simulink model "p1_standalone"  (R2014a)
settings: Solver=ode1  SolverMode=SingleTasking  StartTime=0  StopTime=36000  FixedStep=Ts  RelTol=1e-3
PreLoadFcn:
  | InitModel
  | make
InitFcn:
  | InitModel
  | make
values from neighbouring files (symbols this model uses):
  num = num+MTnum(m)    [Build_MtMuMy.m]
  Ts = 0.002    [DSC_Control_Analysis.m]    (also in DSC_Control_Analysis_Exp.m; DSC_Speed_Control_Analysis.m; EC_params_nissan.m; Ext_MPCPara.m = SSD.Ts)
undefined symbols (not defined in the file or in its folder): den, DiscIntNeverNeededParam, gpsins, gr, hal_filter_den, hal_filter_num, Igain_l, Igain_r, Imax_l, Imax_r, Ioff_l, Ioff_r, KB, Kd, KF, Ki, KJ, Kp, param, sglu
libraries: simulink x5, slrtlib x3, xpcdiamondlib x2, UserBlocks x1
(part 1 of 3)
settings Model: SimulationMode=external  ExtModeArmWhenConnect=off  ExtModeAutoUpdateStatusClock=off  Creator=cgadda  LastModifiedBy=cbeal
settings SolverCC: EnableConcurrentExecution=on
settings DataIOCC: LimitDataPoints=off  SignalLogging=off  DSMLogging=off  TimeSaveName=t  OutputSaveName=y  SignalLoggingName=sigsOut
settings OptimizationCC: BooleanDataType=off  InlineParams=on  InlineInvariantSignals=on  ExpressionDepthLimit=2147483647  FoldNonRolledExpr=off  InitFltsAndDblsToZero=on  EfficientFloat2IntCast=on
settings DebuggingCC: SaveWithParameterizedLinksMsg=none  MergeDetectMultiDrivingBlocksExec=error  SolverPrmCheckMsg=none  MultiTaskDSMMsg=warning  MultiTaskCondExecSysMsg=none  StateNameClashWarn=warning
settings HardwareCC: ProdIntDivRoundTo=Zero  ProdEndianess=LittleEndian  ProdHWDeviceType=Generic->32-bit x86 compatible  TargetIntDivRoundTo=Zero  TargetEndianess=LittleEndian  TargetHWDeviceType=32-bit xPC Target (Intel Pentium)
settings RTWCC: SystemTargetFile=slrt.tlc  TemplateMakefile=slrt_default_tmf  Description=Simulink Real-Time  RTWVerbose=off  ProcessScript=slrt_make_rtw_hook  BuildConfiguration=Faster Runs  IncludeERTFirstTime=on  RTWCustomCompilerOptimizations=\Os
settings SimulinkRealTimeCC: GeneratePreprocessorConditionals=Disable all  EnableShiftOperators=on  RL32LogTETModifier=off  RL32LogBufSizeModifier=31000000  xPCRL32EventNumber=100  xPCisDownloadable=off

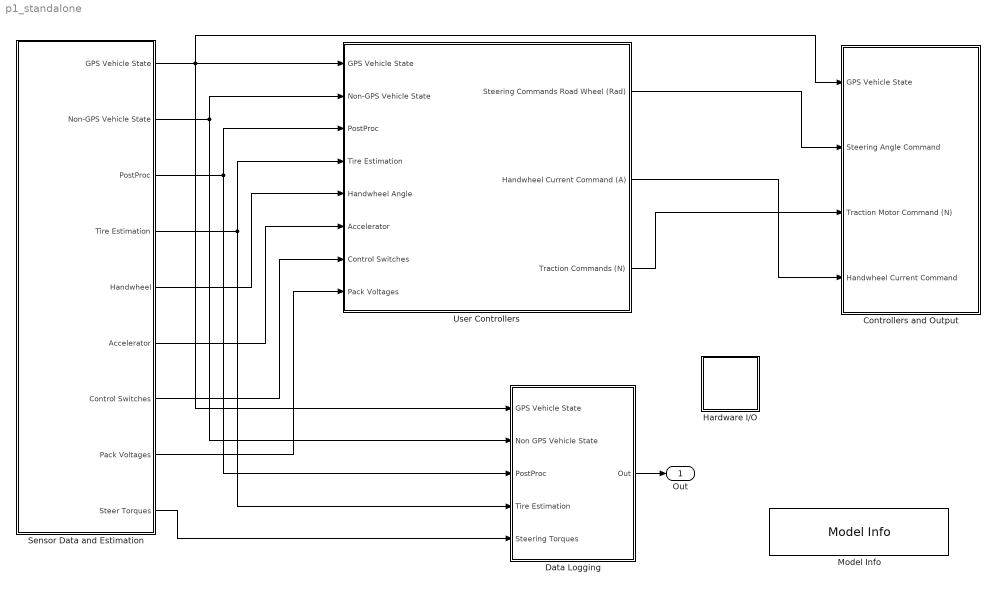
== system p1_standalone ==
  Controllers and Output : Subsystem
  Data Logging : Subsystem
  Hardware I/O : Subsystem  AncestorBlock=HardwareIO/Hardware I//O  mask{OEM4Mode=Velocity (bestvel)}
      mask prompts: OEM4Mode "OEM4 Driver Mode"
      mask init:
      | exist_p1_mdl = sum(strcmp(find_system('p1_standalone', 'searchdepth', 0), 'p1_standalone'));
      | 
      | if (exist_p1_mdl == 1)
      |     set_param('p1_standalone','StopTime','36000');
      |     set_param('p1_standalone','StartTime','0');
      | end
      | 
      | ModeSwitch = [gcs '/Hardware I//O' '/Input' '/OEM4 wgsxyz2enu and status conversion' '/Mode Select'];
      | 
      | if (OEM4Mode == 1)
      |     ModeSelect = 1;
      |     ModeText = 'bestvel';
      |     set_param(ModeSwitch, 'value', '1');
      | elseif (OEM4Mode == 2)
      |     ModeSelect = 0;
      |     ModeText = 'bestxyz';
      |     set_param(ModeSwitch, 'value', '0');
      | end
      mask TypeOptions OEM4Mode: Velocity (bestvel) | Poisition (bestxyz)
      mask Display: disp(['xPC\n' ModeText]);
  Model Info : simulink/Model-Wide Utilities/Model Info  InitialBlockCM=None  BlockCM=None  Frame=off  DisplayStringWithTags=|  HorizontalTextAlignment=Left  LeftAlignmentValue=0.02  SourceBlockDiagram=p1_standalone  TagMaxNumber=20
      | Last saved on: %<LastModificationDate>
      | Save number: %<ModelVersion>
      | Subversion: $Revision: 747 $
  Sensor Data and Estimation : Subsystem
  User Controllers : Subsystem  InitFcn=p1_params SteeringController
  Out : Outport
  wires:
  User Controllers/1(Steering Commands Road Wheel (Rad)) -> Controllers and Output/2(Steering Angle Command)
  Sensor Data and Estimation/1(GPS Vehicle State) -> User Controllers/1(GPS Vehicle State), Controllers and Output/1(GPS Vehicle State), Data Logging/1(GPS Vehicle State)
  Sensor Data and Estimation/2(Non-GPS Vehicle State) -> Data Logging/2(Non GPS Vehicle State), User Controllers/2(Non-GPS Vehicle State)
  Sensor Data and Estimation/3(PostProc) -> User Controllers/3(PostProc), Data Logging/3(PostProc)
  Sensor Data and Estimation/4(Tire Estimation) -> Data Logging/4(Tire Estimation), User Controllers/4(Tire Estimation)
  Data Logging/1(Out) -> Out/1
  User Controllers/3(Traction Commands (N)) -> Controllers and Output/3(Traction Motor Command (N))
  User Controllers/2(Handwheel Current Command (A)) -> Controllers and Output/4(Handwheel Current Command)
  Sensor Data and Estimation/5(Handwheel) -> User Controllers/5(Handwheel Angle)
  Sensor Data and Estimation/6(Accelerator) -> User Controllers/6(Accelerator)
  Sensor Data and Estimation/7(Control Switches) -> User Controllers/7(Control Switches)
  Sensor Data and Estimation/8(Pack Voltages) -> User Controllers/8(Pack Voltages)
  Sensor Data and Estimation/9(Steer Torques) -> Data Logging/5(Steering Torques)

== system p1_standalone/Controllers and Output ==
  GPS Vehicle State : Inport
  Steering Angle Command : Inport  Port=2
  Traction Motor Command (N) : Inport  Port=3
  Handwheel Current Command : Inport  Port=4
  Steering Controller : Subsystem
      mask init:
      | p1_params;
      | SteeringController;
  UI Controller : Subsystem
  tag scope: global_Analog_Meter=global, global_Handwheel_Command=global, global_LED=global, global_Steering_Command=global, global_Traction_Command=global
  wires:
  Steering Angle Command/1 -> Steering Controller/1(Steering Command)
  [global_Handwheel] -> Steering Controller/3(Handwheel Angle)
  [global_Steering] -> Steering Controller/2(Steering Motors)
  [global_Pack_Voltages] -> UI Controller/2(Batteries)
  Steering Controller/1(Current Commands) -> [global_Steering_Command]
  Handwheel Current Command/1 -> [global_Handwheel_Command]
  UI Controller/1(LED) -> [global_LED]
  UI Controller/2(Analog Meter) -> [global_Analog_Meter]
  Traction Motor Command (N)/1 -> [global_Traction_Command]
  GPS Vehicle State/1 -> Steering Controller/4(Vehicle State), UI Controller/1(Vehicle State)
  [global_Cruise_Control] -> UI Controller/3(Switches), Steering Controller/5(switches)

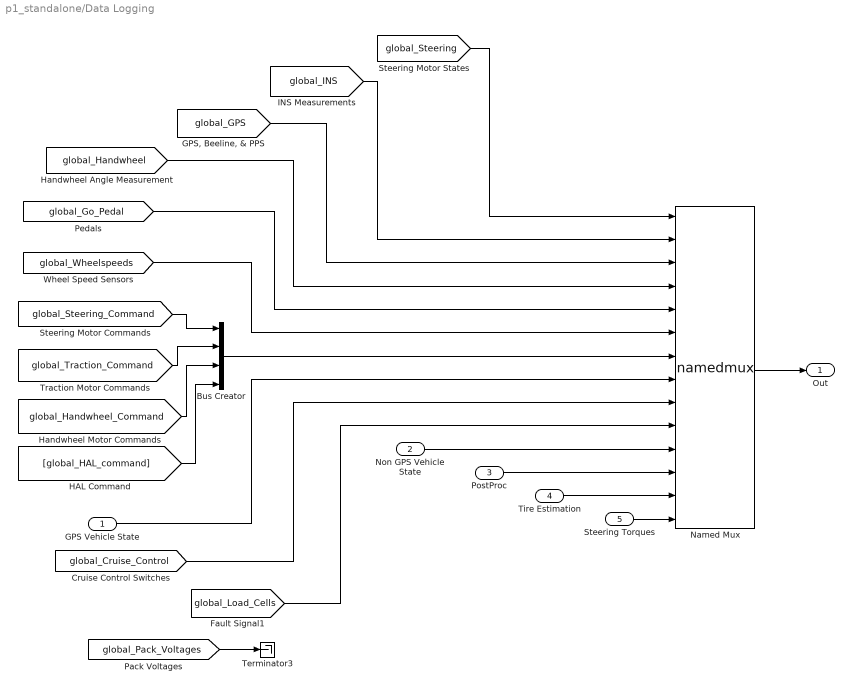
== system p1_standalone/Data Logging ==
  GPS Vehicle State : Inport
  Non GPS Vehicle State : Inport  Port=2
  PostProc : Inport  Port=3
  Tire Estimation : Inport  Port=4
  Steering Torques : Inport  Port=5
  Bus Creator : BusCreator
  Named Mux : S-Function  FunctionName=namedmux  Parameters=inputcount,inputsizes  EnableBusSupport=off  mask{fname=datadesc}
      mask prompts: fname "Data description function name"
      mask help:
      | Combines input signals into a single output vector, according to a structure that provides the names and sizes of each signal.
      |
      | The parameter below should be set to the name of a function which returns a 1xN structure array, where N is the number of input signals.  The structure should contain fields "size" which specifies the width of the input signal, and "name" which specifies its name.
      mask init:
      | desc=eval(fname);
      | %if(class(desc)~='cell')
      | %	error('Incorrect description');
      | %end
      | inputcount=length(desc);
      | if((inputcount<1)|(inputcount>50))
      | 	error('Inappropriate number of inputs.');
      | end
      | 
      | inputsizes=[desc.size];
      | 
      | x=min(inputcount*ones(1,50),1:50);
      mask Display:
      | port_label('input',x(1),desc(x(1)).name);
      | port_label('input',x(2),desc(x(2)).name);
      | port_label('input',x(3),desc(x(3)).name);
      | port_label('input',x(4),desc(x(4)).name);
      | port_label('input',x(5),desc(x(5)).name);
      | port_label('input',x(6),desc(x(6)).name);
      | port_label('input',x(7),desc(x(7)).name);
      | port_label('input',x(8),desc(x(8)).name);
      | port_label('input',x(9),desc(x(9)).name);
      | port_label('input',x(10),desc(x(10)).name);
      | port_label('input',x(11),desc(x(11)).name);
      | port_label('input',x(12),desc(x(12)).name);
      | port_label('input',x(13),desc(x(13)).name);
      | port_label('input',x(14),desc(x(14)).name);
      | port_label('input',x(15),desc(x(15)).name);
      | port_label('input',x(16),desc(x(16)).name);
      | port_label('input',x(17),desc(x(17)).name);
      | port_label('input',x(18),desc(x(18)).name);
      | port_label('input',x(19),desc(x(19)).name);
      | port_label('input',x(20),desc(x(20)).name);
      | port_label('input',x(21),desc(x(21)).name);
      | port_label('input',x(22),desc(x(22)).name);
      | port_label('input',x(23),desc(x(23)).name);
      | port_label('input',x(24),desc(x(24)).name);
      | port_label('input',x(25),desc(x(25)).name);
      | port_label('input',x(26),desc(x(26)).name);
      | port_label('input',x(27),desc(x(27)).name);
      | port_label('input',x(28),desc(x(28)).name);
      | port_label('input',x(29),desc(x(29)).name);
      | port_label('input',x(30),desc(x(30)).name);
  Terminator3 : Terminator
  Out : Outport
  wires:
  GPS Vehicle State/1 -> Named Mux/8
  Named Mux/1 -> Out/1
  [global_Handwheel] -> Named Mux/4
  [global_Steering] -> Named Mux/1
  [global_INS] -> Named Mux/2
  [global_GPS] -> Named Mux/3
  [global_Wheelspeeds] -> Named Mux/6
  [global_Cruise_Control] -> Named Mux/9
  [global_Pack_Voltages] -> Terminator3/1
  [global_Traction_Command] -> Bus Creator/2
  [global_Handwheel_Command] -> Bus Creator/3
  Bus Creator/1 -> Named Mux/7
  [global_Load_Cells] -> Named Mux/10
  [global_Steering_Command] -> Bus Creator/1
  [global_Go_Pedal] -> Named Mux/5
  Non GPS Vehicle State/1 -> Named Mux/11
  PostProc/1 -> Named Mux/12
  Tire Estimation/1 -> Named Mux/13
  Steering Torques/1 -> Named Mux/14
  [global_HAL_command] -> Bus Creator/4

== system p1_standalone/Hardware I//O ==
  Ground : Ground
  Ground1 : Ground
  Input : Subsystem
  Output : Subsystem
  tag scope: global_Cruise_Control=global, global_GPS=global, global_Go_Pedal=global, global_Handwheel=global, global_INS=global, global_Load_Cells=global, global_Pack_Voltages=global, global_Prerecorded_Steering_Command=global, global_Simulation=global, global_Steering=global, global_Wheelspeeds=global
  wires:
  Ground1/1 -> [global_Simulation]
  Ground/1 -> [global_Prerecorded_Steering_Command]
  Input/7(Cruise Control) -> [global_Cruise_Control]
  Input/6(Wheel Speed Sensors) -> [global_Wheelspeeds]
  Input/5(Beeline & GPS) -> [global_GPS]
  Input/4(Go Pedal) -> [global_Go_Pedal]
  Input/3(INS) -> [global_INS]
  Input/2(Steering Motors) -> [global_Steering]
  Input/1(Handwheel) -> [global_Handwheel]
  [global_LED] -> Output/5(Status LED Value)
  [global_Handwheel_Command] -> Output/2(Force Feedback Motor Command)
  [global_Steering_Command] -> Output/1(Steering Motor Commands)
  [global_Analog_Meter] -> Output/4(Analog Meter Command)
  [global_Traction_Command] -> Output/3(Traction Motor Commands (N))
  Input/8(Load Cells) -> [global_Load_Cells]
  Input/9(Pack Voltages) -> [global_Pack_Voltages]

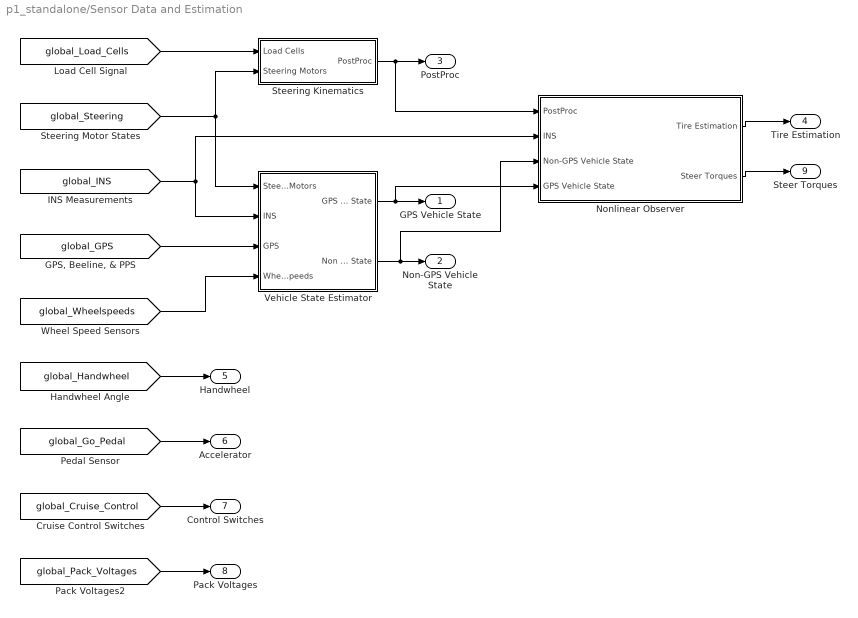
== system p1_standalone/Sensor Data and Estimation ==
  Nonlinear Observer : Subsystem
      mask init:
      | p1_params
      | nissan_steer_lookup_data
      | If_alpha_params
      | [filterb,filtera]=butter(5,0.02);
      | 
      | % dryasphalt = 1;
      | % gravel = 2;
      | % 
      | % AtShoreline = [gcs '/Nonlinear Observer' '/Enable Shoreline Gravel'];
      | % 
      | % % default is dryasphalt
      | % set_param(AtShoreline, 'value', '0');
      | % 
      | % % if gravel selected, make constant AtShoreline = 1
      | % if (roadsurface == gravel)
      | %     set_param(AtShoreline, 'value', '1');
      | % end
      | %
  Steering Kinematics : Subsystem
      mask init:
      | p1_params
      | nissan_steer_lookup_data
  Vehicle State Estimator : Subsystem
      mask init:
      | p1_params;
      | InitVehicleEstimator;
  GPS Vehicle State : Outport
  Non-GPS Vehicle State : Outport  Port=2
  PostProc : Outport  Port=3
  Tire Estimation : Outport  Port=4
  Handwheel : Outport  Port=5
  Accelerator : Outport  Port=6
  Control Switches : Outport  Port=7
  Pack Voltages : Outport  Port=8
  Steer Torques : Outport  Port=9
  wires:
  Vehicle State Estimator/1(GPS Vehicle State) -> GPS Vehicle State/1, Nonlinear Observer/4(GPS Vehicle State)
  Vehicle State Estimator/2(Non GPS Vehicle State) -> Non-GPS Vehicle State/1, Nonlinear Observer/3(Non-GPS Vehicle State)
  Steering Kinematics/1(PostProc) -> PostProc/1, Nonlinear Observer/1(PostProc)
  Nonlinear Observer/1(Tire Estimation) -> Tire Estimation/1
  [global_GPS] -> Vehicle State Estimator/3(GPS)
  [global_INS] -> Vehicle State Estimator/2(INS), Nonlinear Observer/2(INS)
  [global_Steering] -> Steering Kinematics/2(Steering Motors), Vehicle State Estimator/1(Steering Motors)
  [global_Load_Cells] -> Steering Kinematics/1(Load Cells)
  [global_Wheelspeeds] -> Vehicle State Estimator/4(Wheel Speeds)
  [global_Handwheel] -> Handwheel/1
  [global_Go_Pedal] -> Accelerator/1
  [global_Cruise_Control] -> Control Switches/1
  [global_Pack_Voltages] -> Pack Voltages/1
  Nonlinear Observer/2(Steer Torques) -> Steer Torques/1

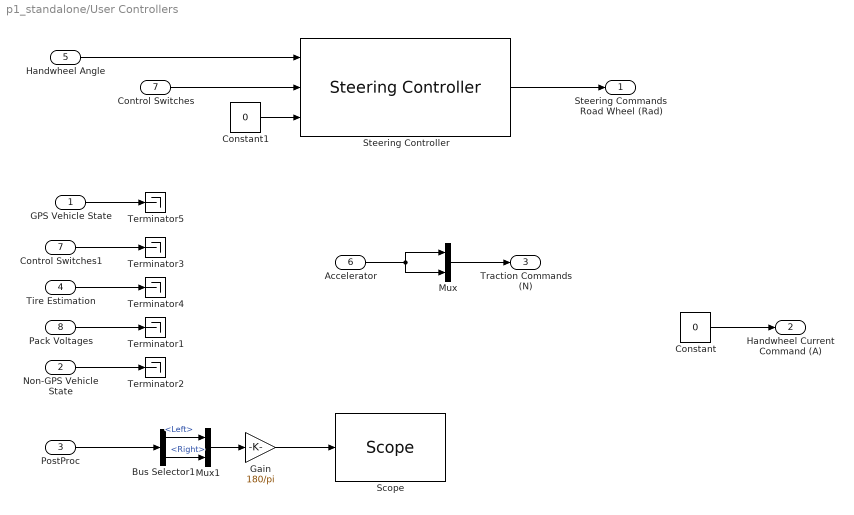
== system p1_standalone/User Controllers ==
  GPS Vehicle State : Inport
  Non-GPS Vehicle State : Inport  Port=2
  PostProc : Inport  Port=3
  Tire Estimation : Inport  Port=4
  Handwheel Angle : Inport  Port=5
  Accelerator : Inport  Port=6
  Control Switches : Inport  Port=7
  Pack Voltages : Inport  Port=8
  Bus Selector1 : BusSelector  OutputSignals=Steer Angles.Left,Steer Angles.Right
  Constant : Constant  Value=0
  Constant1 : Constant  Value=0
  Control Switches1 : InportShadow  Port=7
  Gain : Gain  Gain=180/pi
  Mux : Mux  Inputs=2
  Mux1 : Mux  Inputs=2
  "Scope " : slrtlib/Displays and Logging/Scope   scopeno=2  scopetype=Target  autostart=on  viewmode=Numerical  formatstr='%15.6f'  grid=on  ylimits=[0,0]  nosamples=250  noprepostsamples=0  interleave=1  triggermode=FreeRun  triggersignal=1  trigsignalfromport=off  triggerlevel=0.0  triggerslope=Either  triggerscope=1  triggersample=0  filename=data.dat  mode=Lazy  writesize=512  autorestart=off  dynamicfilemode=off  maxwritefilesize=512*1024^2
  Steering Controller : UserBlocks/Steering Controller  SystemSampleTime=-1
  Terminator{1..5} (5 alike) : Terminator
  Steering Commands Road Wheel (Rad) : Outport
  Handwheel Current Command (A) : Outport  Port=2
  Traction Commands (N) : Outport  Port=3
  wires:
  Non-GPS Vehicle State/1 -> Terminator2/1
  Pack Voltages/1 -> Terminator1/1
  Constant/1 -> Handwheel Current Command (A)/1
  PostProc/1 -> Bus Selector1/1
  Control Switches/1 -> Steering Controller/2
  Handwheel Angle/1 -> Steering Controller/1
  Constant1/1 -> Steering Controller/3
  Mux/1 -> Traction Commands (N)/1
  Accelerator/1 -> Mux/2, Mux/1
  Bus Selector1/1 -> Mux1/1  "<Left>"
  Bus Selector1/2 -> Mux1/2  "<Right>"
  Mux1/1 -> Gain/1
  Steering Controller/1 -> Steering Commands Road Wheel (Rad)/1
  Gain/1 -> "Scope "/1
  Tire Estimation/1 -> Terminator4/1
  Control Switches1/1 -> Terminator3/1
  GPS Vehicle State/1 -> Terminator5/1

== system p1_standalone/Controllers and Output/Steering Controller ==
  Steering Command : Inport
  Steering Motors : Inport  Port=2
  Handwheel Angle : Inport  Port=3
  Vehicle State : Inport  Port=4
  switches : Inport  Port=5
  Bus Selector1 : BusSelector  OutputSignals=Primary
  Bus Selector2 : BusSelector  OutputSignals=Angles
  Bus Selector3 : BusSelector  OutputSignals=Vx
  Bus Selector4 : BusSelector  OutputSignals=Auto-Steer Switch
  Constant : Constant  Value=0
  Demux : Demux  Outputs=2
  Demux1 : Demux  Outputs=2
  LF steering controller : Subsystem
  Mux : Mux  Inputs=2
  Product : Product  SaturateOnIntegerOverflow=on  OutDataTypeStr=Inherit: Same as first input
  RF steering controller : Subsystem
  "Scope " : slrtlib/Displays and Logging/Scope   scopeno=3  scopetype=Target  autostart=on  viewmode=Numerical  formatstr='%15.6f'  grid=on  ylimits=[0,0]  nosamples=250  noprepostsamples=0  interleave=1  triggermode=FreeRun  triggersignal=1  trigsignalfromport=off  triggerlevel=0.0  triggerslope=Either  triggerscope=1  triggersample=0  filename=data.dat  mode=Lazy  writesize=512  autorestart=off  dynamicfilemode=off  maxwritefilesize=512*1024^2
  Steering Geometry & Gearbox Correction : Subsystem
      mask init:
      | p1_params
      | nissan_steer_lookup_data
  standby : Subsystem
  Current Commands : Outport
  wires:
  Vehicle State/1 -> Bus Selector3/1
  Demux1/2 -> RF steering controller/2(actual angle)
  Demux1/1 -> LF steering controller/2(actual angle)
  Demux/1 -> LF steering controller/1(command angle)
  Demux/2 -> RF steering controller/1(command angle)
  RF steering controller/1(current command) -> Mux/2  "Right Current Command"
  Mux/1 -> Product/1
  Steering Motors/1 -> Bus Selector2/1
  Bus Selector2/1 -> Demux1/1  "<Angles>"
  Steering Geometry & Gearbox Correction/1(Shaft Angles) -> Demux/1
  standby/1(Enable) -> Product/2
  Product/1 -> Current Commands/1, "Scope "/1
  Bus Selector3/1 -> standby/2(Speed)  "<Vx>"
  Constant/1 -> RF steering controller/3(aligning moment), LF steering controller/3(aligning moment)
  Steering Command/1 -> Steering Geometry & Gearbox Correction/1(Steer Angles)
  Handwheel Angle/1 -> Bus Selector1/1
  Bus Selector1/1 -> standby/1(Handwheel Angle)  "<Primary>"
  switches/1 -> Bus Selector4/1
  Bus Selector4/1 -> standby/3(autoSteerSwitch)  "<Auto-Steer Switch>"
  LF steering controller/1(current command) -> Mux/1  "Left Current Command"

== system p1_standalone/Controllers and Output/UI Controller ==
  Vehicle State : Inport
  Batteries : Inport  Port=2
  Switches : Inport  Port=3
  Heartbeat Signal : DiscretePulseGenerator  PulseType=Time based  Period=.5  PulseWidth=50
  Speedometer : Subsystem  mask{fsv=25, units=m/s}
      mask prompts: fsv "Full-scale value"
      mask init:
      | unitLabels={'m/s','MPH','KPH'};
      | unitValues={1,2.23693629,3.6};
      | 
      | label=unitLabels{units};
      | scaleFactor=unitValues{units}/fsv;
      mask TypeOptions units: m/s | MPH | KPH
      mask Display: disp(sprintf('%d %s',fsv,label));
  Terminator : Terminator
  Terminator1 : Terminator
  LED : Outport
  Analog Meter : Outport  Port=2
  wires:
  Heartbeat Signal/1 -> LED/1
  Batteries/1 -> Terminator/1
  Vehicle State/1 -> Speedometer/1(Vehicle State)
  Speedometer/1(Meter) -> Analog Meter/1
  Switches/1 -> Terminator1/1

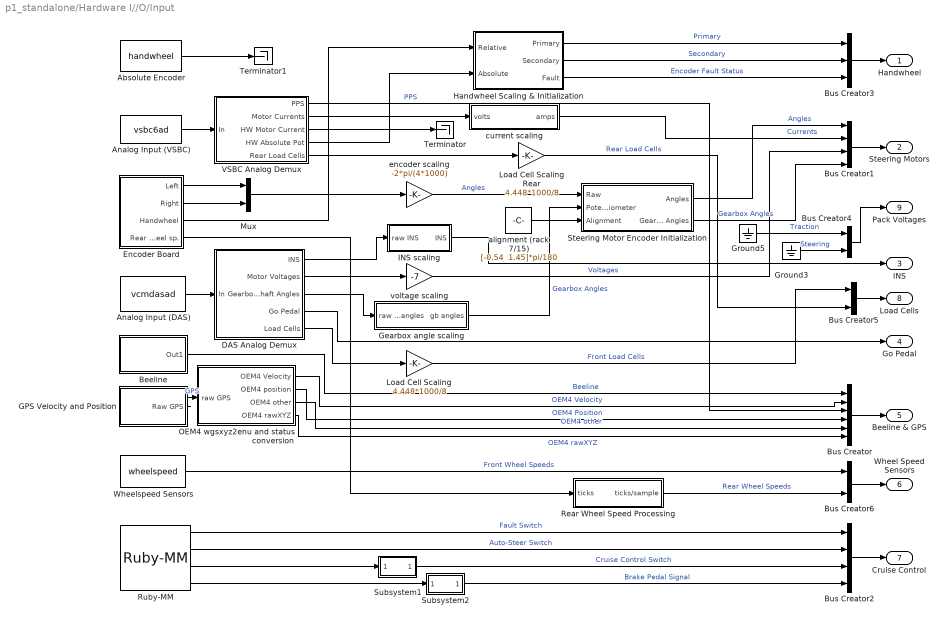
== system p1_standalone/Hardware I//O/Input ==
  Absolute Encoder : S-Function  FunctionName=handwheel  Parameters=Ts  EnableBusSupport=off
  Analog Input (DAS) : S-Function  FunctionName=vcmdasad  Parameters=numChannels, inputVec, sampleTime  EnableBusSupport=off  mask{numChannels=16, inputVec=[4 4 4 4 4 4 4 4 4 4 4 4 4 4 4 4], sampleTime=Ts}
      mask prompts: sampleTime "sample_time"
  Analog Input (VSBC) : S-Function  FunctionName=vsbc6ad  Parameters=numChannels,inpRange,sampTime  EnableBusSupport=off  mask{numChannels=8, inpRange=[4 4 1 4 4 3 3 2], sampTime=Ts}
      mask prompts: numChannels "Number of Channels"; inpRange "Analog Input Range (1: +5; 2: +10; 3: +-5; 4: +-10)"; sampTime "Sampling Time"
  Beeline : Subsystem
      mask Display: disp('beeline');
  Bus Creator : BusCreator  Inputs=6
  Bus Creator1 : BusCreator
  Bus Creator2 : BusCreator
  Bus Creator3 : BusCreator  Inputs=3
  Bus Creator4 : BusCreator  Inputs=2
  Bus Creator5 : BusCreator  Inputs=2
  Bus Creator6 : BusCreator  Inputs=2
  DAS Analog Demux : Subsystem
  Encoder Board : Subsystem
  GPS Velocity and Position : Subsystem
      mask Display: disp('OEM4');
  Gearbox angle scaling : Subsystem
  Ground3 : Ground
  Ground5 : Ground
  Handwheel Scaling & Initialization : Subsystem
  INS scaling : Subsystem
  Load Cell Scaling : Gain  Gain=4.448*1000/8  SaturateOnIntegerOverflow=on  OutDataTypeStr=Inherit: Same as input  ParamDataTypeStr=Inherit: Same as input
  Load Cell Scaling Rear : Gain  Gain=4.448*1000/8  SaturateOnIntegerOverflow=on  OutDataTypeStr=Inherit: Same as input  ParamDataTypeStr=Inherit: Same as input
  Mux : Mux  Inputs=2
  OEM4 wgsxyz2enu and status conversion : Subsystem  AncestorBlock=IOlib/Hardware I//O/Input/INS scaling
  Rear Wheel Speed Processing : Subsystem
  Ruby-MM : xpcdiamondlib/Digital Input/Ruby-MM   channel=[5 6 7 8]  port=A  chip=1  sampletime=Ts  baseaddress=0x300
  Steering Motor Encoder Initialization : Subsystem
      mask init:
      | p1_params
  Subsystem1 : Subsystem
      mask Display: disp('!');
  Subsystem2 : Subsystem
      mask Display: disp('!');
  Terminator : Terminator
  Terminator1 : Terminator
  VSBC Analog Demux : Subsystem
  Wheelspeed Sensors : S-Function  FunctionName=wheelspeed  Parameters=Ts  EnableBusSupport=off
  alignment (rack 7/15) : Constant  Value="[-0.54  1.45]*pi/180"
  current scaling : Subsystem
  encoder scaling : Gain  Gain=-2*pi/(4*1000)  SaturateOnIntegerOverflow=on  OutDataTypeStr=Inherit: Same as input  ParamDataTypeStr=Inherit: Same as input
  voltage scaling : Gain  Gain=-7  SaturateOnIntegerOverflow=on  OutDataTypeStr=Inherit: Same as input  ParamDataTypeStr=Inherit: Same as input
  Handwheel : Outport
  Steering Motors : Outport  Port=2
  INS : Outport  Port=3
  Go Pedal : Outport  Port=4
  Beeline & GPS : Outport  Port=5
  Wheel Speed Sensors : Outport  Port=6
  Cruise Control : Outport  Port=7
  Load Cells : Outport  Port=8
  Pack Voltages : Outport  Port=9
  wires:
  VSBC Analog Demux/4(HW Absolute Pot) -> Handwheel Scaling & Initialization/2(Absolute)
  Handwheel Scaling & Initialization/1(Primary) -> Bus Creator3/1  "Primary"
  OEM4 wgsxyz2enu and status conversion/3(OEM4 other) -> Bus Creator/5  "OEM4 other"
  OEM4 wgsxyz2enu and status conversion/2(OEM4 position) -> Bus Creator/4  "OEM4 Position"
  GPS Velocity and Position/1(Raw GPS) -> OEM4 wgsxyz2enu and status conversion/1(raw GPS)  "GPS"
  OEM4 wgsxyz2enu and status conversion/1(OEM4 Velocity) -> Bus Creator/2  "OEM4 Velocity"
  Ground5/1 -> Bus Creator4/1  "Traction"
  Ruby-MM/1 -> Bus Creator2/1  "Fault Switch"
  Ruby-MM/2 -> Bus Creator2/2  "Auto-Steer Switch"
  Ruby-MM/4 -> Subsystem2/1(In1)
  Ruby-MM/3 -> Subsystem1/1(In1)
  Steering Motor Encoder Initialization/2(Gearbox Angles) -> Bus Creator1/4  "Gearbox Angles"
  alignment (rack 7/15)/1 -> Steering Motor Encoder Initialization/3(Alignment)
  Steering Motor Encoder Initialization/1(Angles) -> Bus Creator1/1  "Angles"
  Handwheel Scaling & Initialization/3(Fault) -> Bus Creator3/3  "Encoder Fault Status"
  encoder scaling/1 -> Steering Motor Encoder Initialization/1(Raw)  "Angles"
  Subsystem2/1(Out1) -> Bus Creator2/4  "Brake Pedal Signal"
  Subsystem1/1(Out1) -> Bus Creator2/3  "Cruise Control Switch"
  Gearbox angle scaling/1(gb angles) -> Steering Motor Encoder Initialization/2(Potentiometer)  "Gearbox Angles"
  DAS Analog Demux/3(Gearbox Shaft Angles) -> Gearbox angle scaling/1(raw gb angles)
  Analog Input (DAS)/1 -> DAS Analog Demux/1(In)
  DAS Analog Demux/1(INS) -> INS scaling/1(raw INS)
  INS scaling/1(INS) -> INS/1
  current scaling/1(amps) -> Bus Creator1/2  "Currents"
  VSBC Analog Demux/2(Motor Currents) -> current scaling/1(volts)
  Bus Creator1/1 -> Steering Motors/1
  Bus Creator/1 -> Beeline & GPS/1
  Beeline/1(Out1) -> Bus Creator/1  "Beeline"
  VSBC Analog Demux/1(PPS) -> Bus Creator/3  "PPS"
  Analog Input (VSBC)/1 -> VSBC Analog Demux/1(In)
  Encoder Board/1(Left) -> Mux/1
  Encoder Board/2(Right) -> Mux/2
  Mux/1 -> encoder scaling/1
  voltage scaling/1 -> Bus Creator1/3  "Voltages"
  DAS Analog Demux/2(Motor Voltages) -> voltage scaling/1
  Bus Creator2/1 -> Cruise Control/1
  DAS Analog Demux/4(Go Pedal) -> Go Pedal/1
  Bus Creator3/1 -> Handwheel/1
  Handwheel Scaling & Initialization/2(Secondary) -> Bus Creator3/2  "Secondary"
  DAS Analog Demux/5(Load Cells) -> Load Cell Scaling/1
  Bus Creator4/1 -> Pack Voltages/1
  Ground3/1 -> Bus Creator4/2  "Steering"
  Encoder Board/3(Handwheel) -> Handwheel Scaling & Initialization/1(Relative)
  VSBC Analog Demux/3(HW Motor Current) -> Terminator/1
  Absolute Encoder/1 -> Terminator1/1
  Load Cell Scaling/1 -> Bus Creator5/1  "Front Load Cells"
  VSBC Analog Demux/5(Rear Load Cells) -> Load Cell Scaling Rear/1
  Load Cell Scaling Rear/1 -> Bus Creator5/2  "Rear Load Cells"
  Bus Creator5/1 -> Load Cells/1
  Wheelspeed Sensors/1 -> Bus Creator6/1  "Front Wheel Speeds"
  Rear Wheel Speed Processing/1(ticks/sample) -> Bus Creator6/2  "Rear Wheel Speeds"
  Encoder Board/4(Rear wheel sp.) -> Rear Wheel Speed Processing/1(ticks)
  Bus Creator6/1 -> Wheel Speed Sensors/1
  OEM4 wgsxyz2enu and status conversion/4(OEM4 rawXYZ) -> Bus Creator/6  "OEM4 rawXYZ"

== system p1_standalone/Hardware I//O/Output ==
  Steering Motor Commands : Inport
  Force Feedback Motor Command : Inport  Port=2
  Traction Motor Commands (N) : Inport  Port=3
  Analog Meter Command : Inport  Port=4
  Status LED Value : Inport  Port=5
  1.0 = full scale : Gain  Gain=9.7  SaturateOnIntegerOverflow=on  OutDataTypeStr=Inherit: Same as input  ParamDataTypeStr=Inherit: Same as input
  ConvertForce2Volt : Subsystem  TreatAsAtomicUnit=on
  Demux : Demux  Outputs=2
  Demux1 : Demux  Outputs=2
  Ground2 : Ground
  "Ruby-MM " : xpcdiamondlib/D//A/Ruby-MM   channel=[1 2 3 4 5 6 7]  range0=+-10  range1=+-10  reset=[1 1 1 1 1 1 1]  initValue=[0 0 0 0 0 0 0]  st=Ts  baseaddress=0x300
  Status LED : S-Function  FunctionName=vsbc8led  EnableBusSupport=off
  amps to volts : Gain  Gain=1/3.96  SaturateOnIntegerOverflow=on  OutDataTypeStr=Inherit: Same as input  ParamDataTypeStr=Inherit: Same as input
  raw signal : Gain  Gain=2  SaturateOnIntegerOverflow=on  OutDataTypeStr=Inherit: Same as input  ParamDataTypeStr=Inherit: Same as input
  saturation : Saturate  UpperLimit=11  LowerLimit=0
  saturation 2 : Saturate  UpperLimit=6  LowerLimit=0  OutDataTypeStr=Inherit: Inherit via back propagation
  saturation1 : Saturate  UpperLimit=2  LowerLimit=-2
  voltage gain : Gain  Gain=7.57/30  SaturateOnIntegerOverflow=on  OutDataTypeStr=Inherit: Same as input  ParamDataTypeStr=Inherit: Same as input
  wires:
  saturation1/1 -> amps to volts/1
  Analog Meter Command/1 -> 1.0 = full scale/1
  Traction Motor Commands (N)/1 -> ConvertForce2Volt/1(ForceDesired)
  Demux1/1 -> "Ruby-MM "/5
  Status LED Value/1 -> Status LED/1
  Demux/1 -> "Ruby-MM "/1
  Demux/2 -> "Ruby-MM "/2
  Ground2/1 -> "Ruby-MM "/4
  1.0 = full scale/1 -> saturation/1
  voltage gain/1 -> Demux/1
  Steering Motor Commands/1 -> voltage gain/1
  Demux1/2 -> "Ruby-MM "/6
  saturation/1 -> "Ruby-MM "/7
  saturation 2/1 -> Demux1/1
  raw signal/1 -> saturation 2/1
  Force Feedback Motor Command/1 -> saturation1/1
  amps to volts/1 -> "Ruby-MM "/3
  ConvertForce2Volt/1(VoltDesired) -> raw signal/1

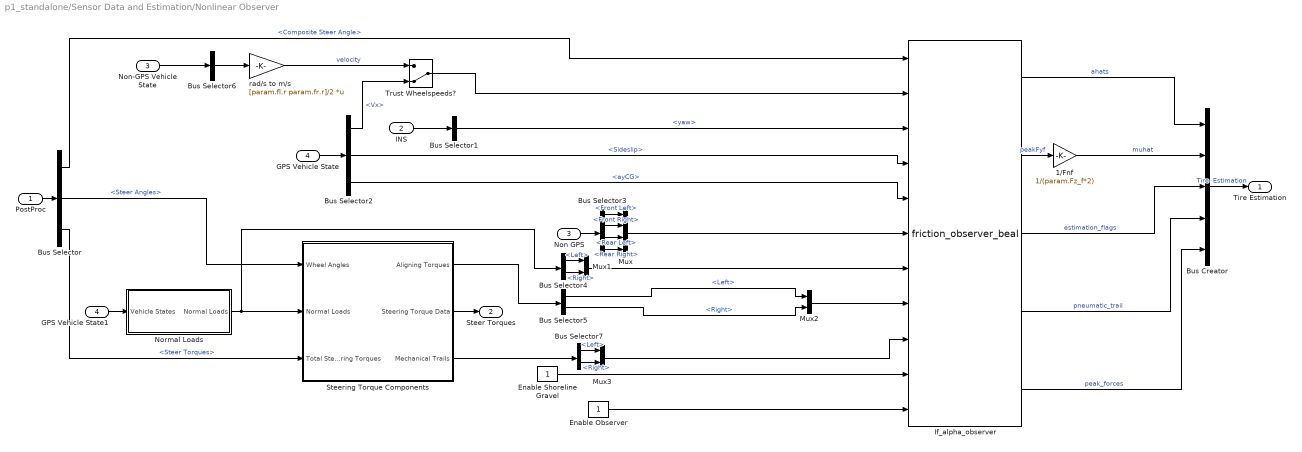
== system p1_standalone/Sensor Data and Estimation/Nonlinear Observer ==
  PostProc : Inport
  INS : Inport  Port=2
  Non-GPS Vehicle State : Inport  Port=3
  GPS Vehicle State : Inport  Port=4
  1/Fnf : Gain  Gain=1/(param.Fz_f*2)
  Bus Creator : BusCreator  Inputs=5
  Bus Selector : BusSelector  OutputSignals=Composite Steer Angle,Steer Angles,Steer Torques
  Bus Selector1 : BusSelector  OutputSignals=yaw
  Bus Selector2 : BusSelector  OutputSignals=Vx,Sideslip,ayCG
  Bus Selector3 : BusSelector  OutputSignals=Wheel Speeds.Front Left,Wheel Speeds.Front Right,Wheel Speeds.Rear Left,Wheel Speeds.Rear Right
  Bus Selector4 : BusSelector  OutputSignals=Left,Right
  Bus Selector5 : BusSelector  OutputSignals=Left,Right
  Bus Selector6 : BusSelector  OutputSignals=Wheel Speeds.Front Left,Wheel Speeds.Front Right  OutputAsBus=on
  Bus Selector7 : BusSelector  OutputSignals=Left,Right
  Enable Observer : Constant
  Enable Shoreline Gravel : Constant
  GPS Vehicle State1 : InportShadow  Port=4
  If_alpha_observer : S-Function  FunctionName=friction_observer_beal  Parameters=Ts, param.a, param.b, param.m, param.Iz, Ifalphaparam.tp0L, Ifalphaparam.tp0R, Ifalphaparam.Caf, Ifalphaparam.Car, Ifalphaparam.Caf_shoreline_sf, Ifalphaparam.Car_shoreline_sf, Ifalphaparam.alphafoffset, Ifalphaparam.alpharoffset, Ifalphaparam.mu_peak_nom, Ifalphaparam.Kaf0, Ifalphaparam.Kaf_sf_Shoreline, Ifalphaparam.Kaf_sf_asphalt, Ifalphaparam.Vfloor, Ifalphaparam.ayfloor, Ifalphaparam.alpha_thres, Ifalphaparam.afhatceil, Ifalphaparam.kappaceil  EnableBusSupport=off
  Mux : Mux
  Mux1 : Mux  Inputs=2
  Mux2 : Mux  Inputs=2
  Mux3 : Mux  Inputs=2
  Non GPS : InportShadow  Port=3
  Normal Loads : Subsystem
      mask init:
      | p1_params
      | nissan_steer_lookup_data
  Steering Torque Components : Subsystem
      mask init:
      | p1_params;
      | nissan_steer_lookup_data;
      | SteeringController;
  Trust Wheelspeeds? : ManualSwitch  CurrentSetting=0
  rad/s to m/s : Gain  Gain=[param.fl.r param.fr.r]/2  Multiplication=Matrix(K*u)
  Tire Estimation : Outport
  Steer Torques : Outport  Port=2
  wires:
  PostProc/1 -> Bus Selector/1
  Bus Creator/1 -> Tire Estimation/1  "Tire  Estimation"
  INS/1 -> Bus Selector1/1
  Non-GPS Vehicle State/1 -> Bus Selector6/1
  rad/s to m/s/1 -> Trust Wheelspeeds?/1  "velocity"
  Bus Selector/1 -> If_alpha_observer/1  "<Composite Steer Angle>"
  Bus Selector1/1 -> If_alpha_observer/3  "<yaw>"
  Bus Selector2/2 -> If_alpha_observer/4  "<Sideslip>"
  Bus Selector2/3 -> If_alpha_observer/5  "<ayCG>"
  Bus Selector/3 -> Steering Torque Components/3(Total Steering Torques)  "<Steer Torques>"
  If_alpha_observer/1 -> Bus Creator/1  "ahats"
  If_alpha_observer/3 -> Bus Creator/3  "estimation_flags"
  If_alpha_observer/2 -> 1/Fnf/1  "peakFyf"
  Bus Selector6/1 -> rad/s to m/s/1
  Trust Wheelspeeds?/1 -> If_alpha_observer/2
  GPS Vehicle State/1 -> Bus Selector2/1
  If_alpha_observer/4 -> Bus Creator/4  "pneumatic_trail"
  Bus Selector2/1 -> Trust Wheelspeeds?/2  "<Vx>"
  Normal Loads/1(Normal Loads) -> Steering Torque Components/2(Normal Loads), Bus Selector4/1
  GPS Vehicle State1/1 -> Normal Loads/1(Vehicle States)
  Steering Torque Components/2(Steering Torque Data) -> Steer Torques/1
  If_alpha_observer/5 -> Bus Creator/5  "peak_forces"
  Enable Shoreline Gravel/1 -> If_alpha_observer/10
  Enable Observer/1 -> If_alpha_observer/11
  Non GPS/1 -> Bus Selector3/1
  Bus Selector3/1 -> Mux/1  "<Front Left>"
  Bus Selector3/2 -> Mux/2  "<Front Right>"
  Bus Selector3/3 -> Mux/3  "<Rear Left>"
  Bus Selector3/4 -> Mux/4  "<Rear Right>"
  Mux/1 -> If_alpha_observer/6
  Bus Selector4/1 -> Mux1/1  "<Left>"
  Bus Selector4/2 -> Mux1/2  "<Right>"
  Mux1/1 -> If_alpha_observer/7
  Bus Selector7/1 -> Mux3/1  "<Left>"
  Bus Selector7/2 -> Mux3/2  "<Right>"
  Steering Torque Components/1(Aligning Torques) -> Bus Selector5/1
  Mux2/1 -> If_alpha_observer/8
  Mux3/1 -> If_alpha_observer/9
  Steering Torque Components/3(Mechanical Trails) -> Bus Selector7/1
  1/Fnf/1 -> Bus Creator/2  "muhat"
  Bus Selector5/1 -> Mux2/1  "<Left>"
  Bus Selector5/2 -> Mux2/2  "<Right>"
  Bus Selector/2 -> Steering Torque Components/1(Wheel Angles)  "<Steer Angles>"

== system p1_standalone/Sensor Data and Estimation/Steering Kinematics ==
  Load Cells : Inport
  Steering Motors : Inport  Port=2
  Bus Creator : BusCreator  Inputs=3
  Bus Selector : BusSelector  OutputSignals=Angles
  Bus Selector1 : BusSelector  OutputSignals=Front Load Cells
  Composite Steer Angle Calculation : Fcn  Expr="atan(1 / (1/tan(u[1]) + param.tw/2/(param.a+param.b)))/2  +  atan(1 / (1/tan(u[2]) - param.tw/2/(param.a+param.b)))/2"
  Steer Torque Calculation : Subsystem
      mask init:
      | p1_params
      | nissan_steer_lookup_data
  Steering Angle Calculation : Subsystem
      mask init:
      | p1_params
      | nissan_steer_lookup_data
  PostProc : Outport
  wires:
  Steering Motors/1 -> Bus Selector/1
  Bus Selector/1 -> Steering Angle Calculation/1(Motor Angles), Steer Torque Calculation/1(Motor Angles)  "<Angles>"
  Steering Angle Calculation/1(Steer Angles) -> Composite Steer Angle Calculation/1, Bus Creator/1  "Steer Angles"
  Composite Steer Angle Calculation/1 -> Bus Creator/2  "Composite Steer Angle"
  Steer Torque Calculation/1(Steer Torques) -> Bus Creator/3  "Steer Torques"
  Bus Creator/1 -> PostProc/1  "PostProc"
  Load Cells/1 -> Bus Selector1/1
  Bus Selector1/1 -> Steer Torque Calculation/2(Load Cells)  "<Front Load Cells>"

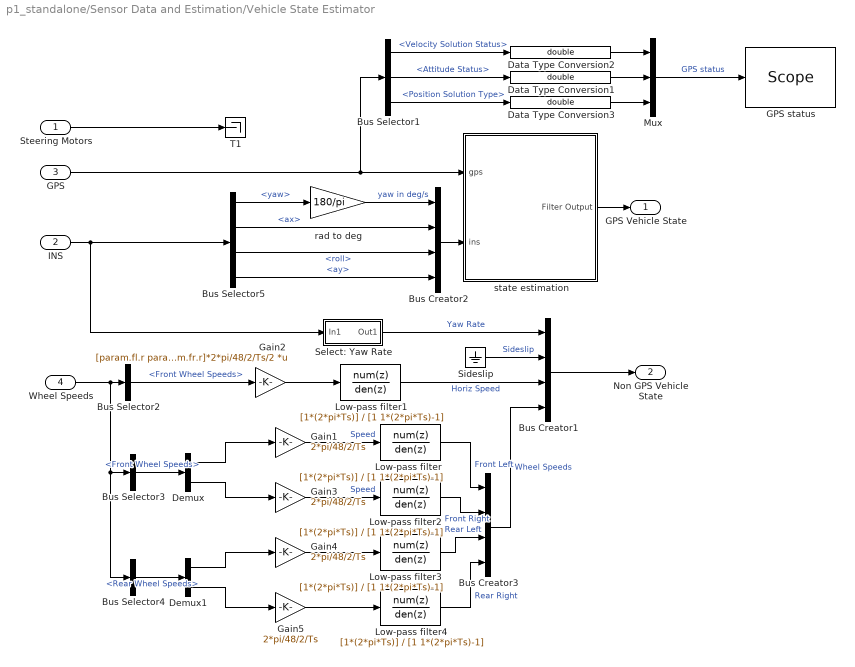
== system p1_standalone/Sensor Data and Estimation/Vehicle State Estimator ==
  Steering Motors : Inport
  INS : Inport  Port=2
  GPS : Inport  Port=3
  Wheel Speeds : Inport  Port=4
  Bus Creator1 : BusCreator
  Bus Creator2 : BusCreator
  Bus Creator3 : BusCreator
  Bus Selector1 : BusSelector  OutputSignals=OEM4 Velocity.Velocity Solution Status,Beeline.Attitude Status,OEM4 Position.Position Solution Type
  Bus Selector2 : BusSelector  OutputSignals=Front Wheel Speeds
  Bus Selector3 : BusSelector  OutputSignals=Front Wheel Speeds
  Bus Selector4 : BusSelector  OutputSignals=Rear Wheel Speeds
  Bus Selector5 : BusSelector  OutputSignals=yaw,ax,roll,ay
  Data Type Conversion1 : DataTypeConversion  OutDataTypeStr=double  RndMeth=Nearest  SaturateOnIntegerOverflow=on
  Data Type Conversion2 : DataTypeConversion  OutDataTypeStr=double  RndMeth=Nearest  SaturateOnIntegerOverflow=on
  Data Type Conversion3 : DataTypeConversion  OutDataTypeStr=double  RndMeth=Nearest  SaturateOnIntegerOverflow=on
  Demux : Demux  Outputs=2
  Demux1 : Demux  Outputs=2
  GPS status : slrtlib/Displays and Logging/Scope   scopeno=1  scopetype=Target  autostart=on  viewmode=Numerical  formatstr='OEM4 Vel (Good=3): %5.3f, BL Att (Good=4): %5.3f, OEM4 Pos (BaseS=5): %5.3f'  grid=on  ylimits=[-10,10]  nosamples=round(1/Ts)  noprepostsamples=0  interleave=1  triggermode=FreeRun  triggersignal=1  trigsignalfromport=off  triggerlevel=0.0  triggerslope=Either  triggerscope=1  triggersample=0  filename=data.dat  mode=Lazy  writesize=512  autorestart=off  dynamicfilemode=off  maxwritefilesize=512*1024^2
  Gain{1,3..5} (4 alike) : Gain  Gain=2*pi/48/2/Ts
  Gain2 : Gain  Gain=[param.fl.r param.fr.r]*2*pi/48/2/Ts/2  Multiplication=Matrix(K*u)
  Low-pass filter{,1..4} (5 alike) : DiscreteTransferFcn  Numerator=[1*(2*pi*Ts)]  Denominator=[1 1*(2*pi*Ts)-1]  SampleTime=Ts
  Mux : Mux  Inputs=3
  Select: Yaw Rate : Subsystem  mask{indices=1, width=6}
      mask prompts: indices "Signal indices"; width "Input width"
      mask init:
      | ic=length(indices);
      | 
      | K=zeros(ic,width);
      | 
      | for ii=1:ic,
      | 	K(ii,indices(ii))=1;
      | end
      mask Display: disp(indices)
  Sideslip : Ground
  T1 : Terminator
  rad to deg : Gain  Gain=180/pi
  state estimation : Subsystem
      mask init:
      | InitModel;
      | ssest_params;
  GPS Vehicle State : Outport
  Non GPS Vehicle State : Outport  Port=2
  wires:
  INS/1 -> Bus Selector5/1, Select: Yaw Rate/1(In1)
  Steering Motors/1 -> T1/1
  Sideslip/1 -> Bus Creator1/2  "Sideslip"
  Bus Creator1/1 -> Non GPS Vehicle State/1
  Bus Creator2/1 -> state estimation/2(ins)
  Bus Selector5/2 -> Bus Creator2/2  "<ax>"
  Bus Selector5/3 -> Bus Creator2/3  "<roll>"
  Bus Selector5/4 -> Bus Creator2/4  "<ay>"
  rad to deg/1 -> Bus Creator2/1  "yaw in deg/s"
  Bus Selector5/1 -> rad to deg/1  "<yaw>"
  Select: Yaw Rate/1(Out1) -> Bus Creator1/1  "Yaw Rate"
  Low-pass filter1/1 -> Bus Creator1/3  "Horiz Speed"
  GPS/1 -> state estimation/1(gps), Bus Selector1/1
  state estimation/1(Filter Output) -> GPS Vehicle State/1
  Bus Selector1/1 -> Data Type Conversion2/1  "<Velocity Solution Status>"
  Bus Selector1/2 -> Data Type Conversion1/1  "<Attitude Status>"
  Bus Selector1/3 -> Data Type Conversion3/1  "<Position Solution Type>"
  Mux/1 -> GPS status/1  "GPS status"
  Data Type Conversion2/1 -> Mux/1
  Data Type Conversion1/1 -> Mux/2
  Data Type Conversion3/1 -> Mux/3
  Wheel Speeds/1 -> Bus Selector2/1, Bus Selector3/1, Bus Selector4/1
  Gain1/1 -> Low-pass filter/1  "Speed"
  Bus Selector2/1 -> Gain2/1  "<Front Wheel Speeds>"
  Gain2/1 -> Low-pass filter1/1
  Gain3/1 -> Low-pass filter2/1  "Speed"
  Bus Creator3/1 -> Bus Creator1/4  "Wheel Speeds"
  Low-pass filter/1 -> Bus Creator3/1  "Front Left"
  Low-pass filter2/1 -> Bus Creator3/2  "Front Right"
  Bus Selector3/1 -> Demux/1  "<Front Wheel Speeds>"
  Demux/1 -> Gain1/1
  Demux/2 -> Gain3/1
  Bus Selector4/1 -> Demux1/1  "<Rear Wheel Speeds>"
  Demux1/1 -> Gain4/1
  Demux1/2 -> Gain5/1
  Gain4/1 -> Low-pass filter3/1
  Gain5/1 -> Low-pass filter4/1
  Low-pass filter4/1 -> Bus Creator3/4  "Rear Right"
  Low-pass filter3/1 -> Bus Creator3/3  "Rear Left"

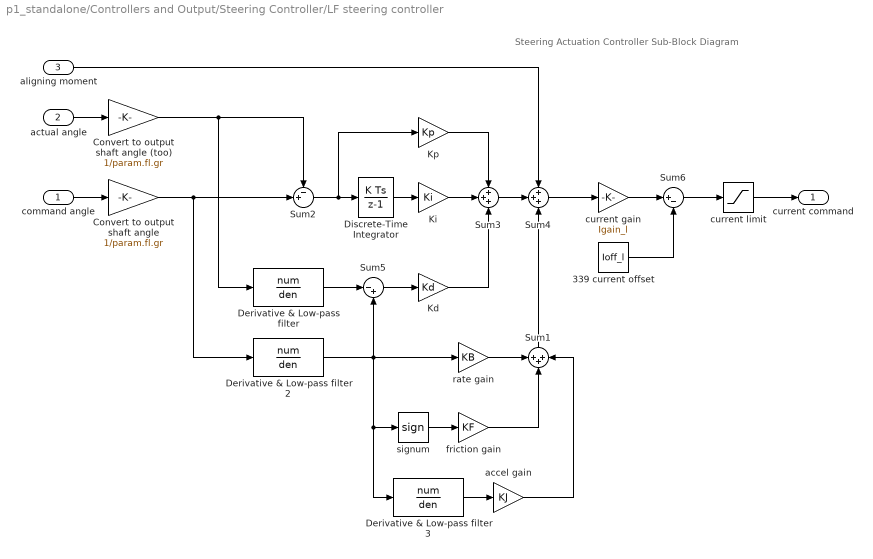
== system p1_standalone/Controllers and Output/Steering Controller/LF steering controller ==
  note: Steering Actuation Controller Sub-Block Diagram
  command angle : Inport
  actual angle : Inport  Port=2
  aligning moment : Inport  Port=3
  339 current offset : Constant  Value=Ioff_l
  Convert to output shaft angle : Gain  Gain=1/param.fl.gr  SaturateOnIntegerOverflow=on  OutDataTypeStr=Inherit: Same as input  ParamDataTypeStr=Inherit: Same as input
  Convert to output shaft angle (too) : Gain  Gain=1/param.fl.gr  SaturateOnIntegerOverflow=on  OutDataTypeStr=Inherit: Same as input  ParamDataTypeStr=Inherit: Same as input
  Derivative & Low-pass filter : DiscreteFilter  Numerator=num  Denominator=den  SampleTime=Ts
  Derivative & Low-pass filter 2 : DiscreteFilter  Numerator=num  Denominator=den  SampleTime=Ts
  Derivative & Low-pass filter 3 : DiscreteFilter  Numerator=num  Denominator=den  SampleTime=Ts
  Discrete-Time Integrator : DiscreteIntegrator  SampleTime=Ts  ICPrevOutput=DiscIntNeverNeededParam  ICPrevScaledInput=DiscIntNeverNeededParam
  Kd : Gain  Gain=Kd  SaturateOnIntegerOverflow=on  OutDataTypeStr=Inherit: Same as input  ParamDataTypeStr=Inherit: Same as input
  Ki : Gain  Gain=Ki  SaturateOnIntegerOverflow=on  OutDataTypeStr=Inherit: Same as input  ParamDataTypeStr=Inherit: Same as input
  Kp : Gain  Gain=Kp  SaturateOnIntegerOverflow=on  OutDataTypeStr=Inherit: Same as input  ParamDataTypeStr=Inherit: Same as input
  Sum1 : Sum  Inputs=+++  SaturateOnIntegerOverflow=on  InputSameDT=on  OutDataTypeStr=Inherit: Same as first input
  Sum2 : Sum  Inputs=-+|  SaturateOnIntegerOverflow=on  InputSameDT=on  OutDataTypeStr=Inherit: Same as first input
  Sum3 : Sum  Inputs=+++  SaturateOnIntegerOverflow=on  InputSameDT=on  OutDataTypeStr=Inherit: Same as first input
  Sum4 : Sum  Inputs=+++  SaturateOnIntegerOverflow=on  InputSameDT=on  OutDataTypeStr=Inherit: Same as first input
  Sum5 : Sum  Inputs=|-+  SaturateOnIntegerOverflow=on  InputSameDT=on  OutDataTypeStr=Inherit: Same as first input
  Sum6 : Sum  Inputs=|+-  SaturateOnIntegerOverflow=on  InputSameDT=on  OutDataTypeStr=Inherit: Same as first input
  accel gain : Gain  Gain=KJ  SaturateOnIntegerOverflow=on  OutDataTypeStr=Inherit: Same as input  ParamDataTypeStr=Inherit: Same as input
  current gain : Gain  Gain=Igain_l  SaturateOnIntegerOverflow=on  OutDataTypeStr=Inherit: Same as input  ParamDataTypeStr=Inherit: Same as input
  current limit : Saturate  UpperLimit=Imax_l  LowerLimit=-Imax_l
  friction gain : Gain  Gain=KF  SaturateOnIntegerOverflow=on  OutDataTypeStr=Inherit: Same as input  ParamDataTypeStr=Inherit: Same as input
  rate gain : Gain  Gain=KB  SaturateOnIntegerOverflow=on  OutDataTypeStr=Inherit: Same as input  ParamDataTypeStr=Inherit: Same as input
  signum : Signum
  current command : Outport
  wires:
  Sum2/1 -> Kp/1, Discrete-Time Integrator/1
  Discrete-Time Integrator/1 -> Ki/1
  Kp/1 -> Sum3/1
  Ki/1 -> Sum3/2
  Sum5/1 -> Kd/1
  Kd/1 -> Sum3/3
  signum/1 -> friction gain/1
  rate gain/1 -> Sum1/1
  friction gain/1 -> Sum1/2
  Sum4/1 -> current gain/1
  Sum3/1 -> Sum4/2
  Sum1/1 -> Sum4/3
  accel gain/1 -> Sum1/3
  aligning moment/1 -> Sum4/1
  command angle/1 -> Convert to output shaft angle/1
  Derivative & Low-pass filter 3/1 -> accel gain/1
  Derivative & Low-pass filter 2/1 -> rate gain/1, Sum5/2, signum/1, Derivative & Low-pass filter 3/1
  current gain/1 -> Sum6/1
  339 current offset/1 -> Sum6/2
  actual angle/1 -> Convert to output shaft angle (too)/1
  Convert to output shaft angle (too)/1 -> Derivative & Low-pass filter/1, Sum2/1
  Derivative & Low-pass filter/1 -> Sum5/1
  Convert to output shaft angle/1 -> Derivative & Low-pass filter 2/1, Sum2/2
  Sum6/1 -> current limit/1
  current limit/1 -> current command/1

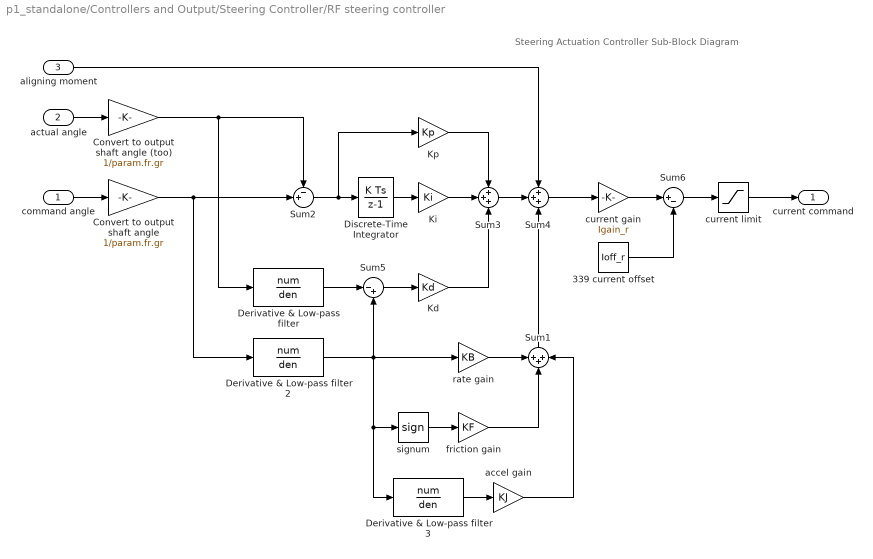
== system p1_standalone/Controllers and Output/Steering Controller/RF steering controller ==
  note: Steering Actuation Controller Sub-Block Diagram
  command angle : Inport
  actual angle : Inport  Port=2
  aligning moment : Inport  Port=3
  339 current offset : Constant  Value=Ioff_r
  Convert to output shaft angle : Gain  Gain=1/param.fr.gr  SaturateOnIntegerOverflow=on  OutDataTypeStr=Inherit: Same as input  ParamDataTypeStr=Inherit: Same as input
  Convert to output shaft angle (too) : Gain  Gain=1/param.fr.gr  SaturateOnIntegerOverflow=on  OutDataTypeStr=Inherit: Same as input  ParamDataTypeStr=Inherit: Same as input
  Derivative & Low-pass filter : DiscreteFilter  Numerator=num  Denominator=den  SampleTime=Ts
  Derivative & Low-pass filter 2 : DiscreteFilter  Numerator=num  Denominator=den  SampleTime=Ts
  Derivative & Low-pass filter 3 : DiscreteFilter  Numerator=num  Denominator=den  SampleTime=Ts
  Discrete-Time Integrator : DiscreteIntegrator  SampleTime=Ts  ICPrevOutput=DiscIntNeverNeededParam  ICPrevScaledInput=DiscIntNeverNeededParam
  Kd : Gain  Gain=Kd  SaturateOnIntegerOverflow=on  OutDataTypeStr=Inherit: Same as input  ParamDataTypeStr=Inherit: Same as input
  Ki : Gain  Gain=Ki  SaturateOnIntegerOverflow=on  OutDataTypeStr=Inherit: Same as input  ParamDataTypeStr=Inherit: Same as input
  Kp : Gain  Gain=Kp  SaturateOnIntegerOverflow=on  OutDataTypeStr=Inherit: Same as input  ParamDataTypeStr=Inherit: Same as input
  Sum1 : Sum  Inputs=+++  SaturateOnIntegerOverflow=on  InputSameDT=on  OutDataTypeStr=Inherit: Same as first input
  Sum2 : Sum  Inputs=-+|  SaturateOnIntegerOverflow=on  InputSameDT=on  OutDataTypeStr=Inherit: Same as first input
  Sum3 : Sum  Inputs=+++  SaturateOnIntegerOverflow=on  InputSameDT=on  OutDataTypeStr=Inherit: Same as first input
  Sum4 : Sum  Inputs=+++  SaturateOnIntegerOverflow=on  InputSameDT=on  OutDataTypeStr=Inherit: Same as first input
  Sum5 : Sum  Inputs=|-+  SaturateOnIntegerOverflow=on  InputSameDT=on  OutDataTypeStr=Inherit: Same as first input
  Sum6 : Sum  Inputs=|+-  SaturateOnIntegerOverflow=on  InputSameDT=on  OutDataTypeStr=Inherit: Same as first input
  accel gain : Gain  Gain=KJ  SaturateOnIntegerOverflow=on  OutDataTypeStr=Inherit: Same as input  ParamDataTypeStr=Inherit: Same as input
  current gain : Gain  Gain=Igain_r  SaturateOnIntegerOverflow=on  OutDataTypeStr=Inherit: Same as input  ParamDataTypeStr=Inherit: Same as input
  current limit : Saturate  UpperLimit=Imax_r  LowerLimit=-Imax_r
  friction gain : Gain  Gain=KF  SaturateOnIntegerOverflow=on  OutDataTypeStr=Inherit: Same as input  ParamDataTypeStr=Inherit: Same as input
  rate gain : Gain  Gain=KB  SaturateOnIntegerOverflow=on  OutDataTypeStr=Inherit: Same as input  ParamDataTypeStr=Inherit: Same as input
  signum : Signum
  current command : Outport
  wires:
  current limit/1 -> current command/1
  Convert to output shaft angle/1 -> Derivative & Low-pass filter 2/1, Sum2/2
  Derivative & Low-pass filter/1 -> Sum5/1
  Convert to output shaft angle (too)/1 -> Derivative & Low-pass filter/1, Sum2/1
  actual angle/1 -> Convert to output shaft angle (too)/1
  Sum6/1 -> current limit/1
  339 current offset/1 -> Sum6/2
  current gain/1 -> Sum6/1
  Derivative & Low-pass filter 2/1 -> Derivative & Low-pass filter 3/1, signum/1, Sum5/2, rate gain/1
  Derivative & Low-pass filter 3/1 -> accel gain/1
  command angle/1 -> Convert to output shaft angle/1
  aligning moment/1 -> Sum4/1
  accel gain/1 -> Sum1/3
  Sum1/1 -> Sum4/3
  Sum3/1 -> Sum4/2
  Sum4/1 -> current gain/1
  friction gain/1 -> Sum1/2
  rate gain/1 -> Sum1/1
  signum/1 -> friction gain/1
  Kd/1 -> Sum3/3
  Sum5/1 -> Kd/1
  Ki/1 -> Sum3/2
  Kp/1 -> Sum3/1
  Discrete-Time Integrator/1 -> Ki/1
  Sum2/1 -> Discrete-Time Integrator/1, Kp/1

== system p1_standalone/Controllers and Output/Steering Controller/Steering Geometry & Gearbox Correction ==
  Steer Angles : Inport
  Demux : Demux  Outputs=2
  Left Steer Angle Look-up : Lookup_n-D  NumberOfTableDimensions=1  BreakpointsForDimension1=sglu.fl.sa  Table=sglu.fl.ma  InternalRulePriority=Speed  SaturateOnIntegerOverflow=on  InputSameDT=on
  Left Steering Ratio : Gain  Gain=param.fl.gr  SaturateOnIntegerOverflow=on  OutDataTypeStr=Inherit: Same as input  ParamDataTypeStr=Inherit: Same as input
  Mux4 : Mux  Inputs=2
  Right Steer Angle Look-up : Lookup_n-D  NumberOfTableDimensions=1  BreakpointsForDimension1=sglu.fr.sa  Table=sglu.fr.ma  InternalRulePriority=Speed  SaturateOnIntegerOverflow=on  InputSameDT=on
  Right Steering Ratio : Gain  Gain=param.fr.gr  SaturateOnIntegerOverflow=on  OutDataTypeStr=Inherit: Same as input  ParamDataTypeStr=Inherit: Same as input
  Shaft Angles : Outport
  wires:
  Steer Angles/1 -> Demux/1
  Demux/1 -> Left Steer Angle Look-up/1
  Demux/2 -> Right Steer Angle Look-up/1
  Left Steer Angle Look-up/1 -> Left Steering Ratio/1
  Right Steer Angle Look-up/1 -> Right Steering Ratio/1
  Left Steering Ratio/1 -> Mux4/1
  Right Steering Ratio/1 -> Mux4/2
  Mux4/1 -> Shaft Angles/1

== system p1_standalone/Controllers and Output/Steering Controller/standby ==
  Handwheel Angle : Inport
  Speed : Inport  Port=2
  autoSteerSwitch : Inport  Port=3
  Derivative & Low-pass filter : DiscreteFilter  Numerator=num  Denominator=den  SampleTime=Ts
  Enable Controller : S-Function  FunctionName=enable  Parameters=timeout,delay,Ts  EnableBusSupport=off  mask{timeout=20000, delay=.5}
      mask prompts: timeout "Inactivity timeout period"; delay "Startup delay"
      mask Display:
      | port_label('input',1,'Angle');
      | port_label('input',2,'Rate');
      | port_label('input',3,'Speed');
      | port_label('input',4,'Switch');
      | port_label('output',1,'Enable');
  filter : DiscreteFilter  Numerator=[2*2*pi*Ts]  Denominator=[1 2*2*pi*Ts-1]  SampleTime=Ts
  filter1 : DiscreteFilter  Numerator=[0.5*2*pi*Ts]  Denominator=[1 0.5*2*pi*Ts-1]  SampleTime=Ts
  Enable : Outport
  wires:
  filter1/1 -> Enable/1
  Enable Controller/1 -> filter1/1
  Handwheel Angle/1 -> Enable Controller/1, Derivative & Low-pass filter/1
  Derivative & Low-pass filter/1 -> filter/1
  filter/1 -> Enable Controller/2
  Speed/1 -> Enable Controller/3
  autoSteerSwitch/1 -> Enable Controller/4

== system p1_standalone/Controllers and Output/UI Controller/Speedometer ==
  Vehicle State : Inport
  Bus Selector1 : BusSelector  OutputSignals=Vx
  Gain : Gain  Gain=scaleFactor  SaturateOnIntegerOverflow=on  OutDataTypeStr=Inherit: Same as input  ParamDataTypeStr=Inherit: Same as input
  Meter : Outport
  wires:
  Bus Selector1/1 -> Gain/1  "<Vx>"
  Vehicle State/1 -> Bus Selector1/1
  Gain/1 -> Meter/1

== system p1_standalone/Hardware I//O/Input/Beeline ==
  Beeline : S-Function  FunctionName=beeline  Parameters=Ts  EnableBusSupport=off
  Bus Creator1 : BusCreator  Inputs=10
  Demux : Demux  Outputs=10
  Out1 : Outport
  wires:
  Beeline/1 -> Demux/1
  Bus Creator1/1 -> Out1/1
  Demux/1 -> Bus Creator1/1  "UTC 1"
  Demux/2 -> Bus Creator1/2  "Yaw Angle"
  Demux/3 -> Bus Creator1/3  "Roll Angle"
  Demux/4 -> Bus Creator1/4  "Attitude Status"
  Demux/5 -> Bus Creator1/5  "UTC 2"
  Demux/6 -> Bus Creator1/6  "Latency"
  Demux/7 -> Bus Creator1/7  "Horizontal Speed"
  Demux/8 -> Bus Creator1/8  "Direction"
  Demux/9 -> Bus Creator1/9  "Vertical Speed"
  Demux/10 -> Bus Creator1/10  "Velocity Status"

== system p1_standalone/Hardware I//O/Input/DAS Analog Demux ==
  In : Inport
  Demux : Demux  Outputs=16
  Mux : Mux  Inputs=9
  Mux1 : Mux  Inputs=2
  Mux2 : Mux  Inputs=2
  Mux3 : Mux  Inputs=2
  INS : Outport
  Motor Voltages : Outport  Port=2
  Gearbox Shaft Angles : Outport  Port=3
  Go Pedal : Outport  Port=4
  Load Cells : Outport  Port=5
  wires:
  Demux/12 -> Mux3/1
  Demux/11 -> Mux3/2
  Mux2/1 -> Gearbox Shaft Angles/1
  In/1 -> Demux/1
  Demux/1 -> Mux/1
  Demux/3 -> Mux/3
  Demux/4 -> Mux/4
  Demux/5 -> Mux/5
  Demux/6 -> Mux/6
  Demux/7 -> Mux/7
  Demux/8 -> Mux/8
  Demux/9 -> Mux/9
  Mux/1 -> INS/1
  Mux1/1 -> Motor Voltages/1
  Demux/13 -> Mux1/1
  Demux/14 -> Mux1/2
  Demux/2 -> Mux/2
  Demux/15 -> Mux2/1
  Demux/16 -> Mux2/2
  Mux3/1 -> Load Cells/1
  Demux/10 -> Go Pedal/1

== system p1_standalone/Hardware I//O/Input/Encoder Board ==
  Mux : Mux  Inputs=2
  "encoder board " : S-Function  FunctionName=UltimateEncoder  Parameters=TSamp,NC,BA,[R1 R2 R3 R4 R5 R6 ]  EnableBusSupport=off  mask{TSamp=Ts, BA=528, NC=5, R1=on, R2=on, R3=on, R4=off, R5=off, R6=off}
      mask prompts: TSamp "Sampling Rate"; BA "Base Adress (Base 10)"; NC "Number of Channels"; R1 "Unwrap Channel 1"; R2 "Unwrap Channel 2"; R3 "Unwrap Channel 3"; R4 "Unwrap Channel 4"; R5 "Unwrap Channel 5"; R6 "Unwrap Channel 6"
  reset : Constant  Value=[1 1 1 0 0]
  Left : Outport
  Right : Outport  Port=2
  Handwheel : Outport  Port=3
  Rear wheel sp. : Outport  Port=4
  wires:
  "encoder board "/2 -> Right/1
  "encoder board "/1 -> Left/1
  reset/1 -> "encoder board "/1
  "encoder board "/3 -> Handwheel/1
  "encoder board "/4 -> Mux/1
  "encoder board "/5 -> Mux/2
  Mux/1 -> Rear wheel sp./1
